simulink model "TST_AirCtl_Gov"  (R2016b)
settings: Solver=FixedStepDiscrete  StartTime=0.0  StopTime=simTime  FixedStep=sampleTime  RelTol=1e-3
values from neighbouring files (symbols this model uses):
  testCase = 1    [initTST_AirCtl_Gov_001.m]
libraries: simulink x6, UnitTest_Lib x4
settings Model: Creator=zhulinfeng  LastModifiedBy=zhulinfeng
settings DebuggingCC: SignalRangeChecking=error

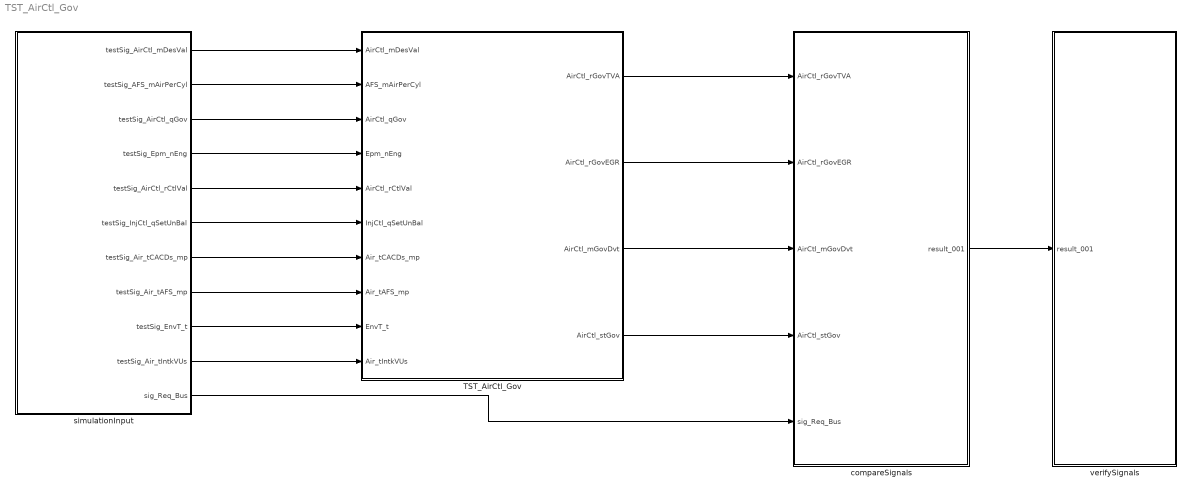
== system TST_AirCtl_Gov ==
  TST_AirCtl_Gov : Subsystem
  compareSignals : Subsystem
  simulationInput : Subsystem
  verifySignals : Subsystem
  wires:
  simulationInput/1(testSig_AirCtl_mDesVal) -> TST_AirCtl_Gov/1(AirCtl_mDesVal)
  simulationInput/2(testSig_AFS_mAirPerCyl) -> TST_AirCtl_Gov/2(AFS_mAirPerCyl)
  simulationInput/3(testSig_AirCtl_qGov) -> TST_AirCtl_Gov/3(AirCtl_qGov)
  simulationInput/4(testSig_Epm_nEng) -> TST_AirCtl_Gov/4(Epm_nEng)
  simulationInput/5(testSig_AirCtl_rCtlVal) -> TST_AirCtl_Gov/5(AirCtl_rCtlVal)
  simulationInput/6(testSig_InjCtl_qSetUnBal) -> TST_AirCtl_Gov/6(InjCtl_qSetUnBal)
  simulationInput/7(testSig_Air_tCACDs_mp) -> TST_AirCtl_Gov/7(Air_tCACDs_mp)
  simulationInput/8(testSig_Air_tAFS_mp) -> TST_AirCtl_Gov/8(Air_tAFS_mp)
  simulationInput/9(testSig_EnvT_t) -> TST_AirCtl_Gov/9(EnvT_t)
  simulationInput/10(testSig_Air_tIntkVUs) -> TST_AirCtl_Gov/10(Air_tIntkVUs)
  TST_AirCtl_Gov/1(AirCtl_rGovTVA) -> compareSignals/1(AirCtl_rGovTVA)
  TST_AirCtl_Gov/2(AirCtl_rGovEGR) -> compareSignals/2(AirCtl_rGovEGR)
  TST_AirCtl_Gov/3(AirCtl_mGovDvt) -> compareSignals/3(AirCtl_mGovDvt)
  TST_AirCtl_Gov/4(AirCtl_stGov) -> compareSignals/4(AirCtl_stGov)
  simulationInput/11(sig_Req_Bus) -> compareSignals/5(sig_Req_Bus)
  compareSignals/1(result_001) -> verifySignals/1(result_001)

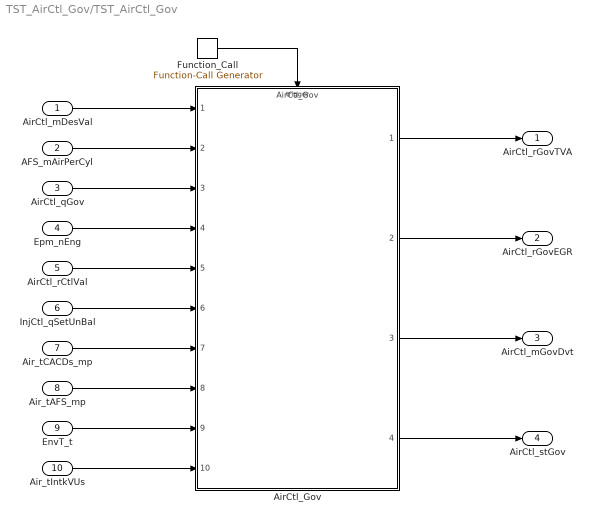
== system TST_AirCtl_Gov/TST_AirCtl_Gov ==
  AirCtl_mDesVal : Inport
  AFS_mAirPerCyl : Inport  Port=2
  AirCtl_qGov : Inport  Port=3
  Epm_nEng : Inport  Port=4
  AirCtl_rCtlVal : Inport  Port=5
  InjCtl_qSetUnBal : Inport  Port=6
  Air_tCACDs_mp : Inport  Port=7
  Air_tAFS_mp : Inport  Port=8
  EnvT_t : Inport  Port=9
  Air_tIntkVUs : Inport  Port=10
  AirCtl_Gov : ModelReference  ModelNameDialog=AirCtl_Gov  SimulationMode=Normal  ModelReferenceVersion=1.96  TriggerPortName=function  TriggerPortTriggerType=function-call  TriggerPortStatesWhenEnabling=held
  Function_Call : simulink/Ports & Subsystems/Function-Call Generator  sample_time=sampleTime  numberOfIterations=1
  AirCtl_rGovTVA : Outport
  AirCtl_rGovEGR : Outport  Port=2
  AirCtl_mGovDvt : Outport  Port=3
  AirCtl_stGov : Outport  Port=4
  wires:
  Function_Call/1 -> AirCtl_Gov/Trigger
  AirCtl_mDesVal/1 -> AirCtl_Gov/1
  AFS_mAirPerCyl/1 -> AirCtl_Gov/2
  AirCtl_qGov/1 -> AirCtl_Gov/3
  Epm_nEng/1 -> AirCtl_Gov/4
  AirCtl_rCtlVal/1 -> AirCtl_Gov/5
  InjCtl_qSetUnBal/1 -> AirCtl_Gov/6
  Air_tCACDs_mp/1 -> AirCtl_Gov/7
  Air_tAFS_mp/1 -> AirCtl_Gov/8
  EnvT_t/1 -> AirCtl_Gov/9
  Air_tIntkVUs/1 -> AirCtl_Gov/10
  AirCtl_Gov/1 -> AirCtl_rGovTVA/1
  AirCtl_Gov/2 -> AirCtl_rGovEGR/1
  AirCtl_Gov/3 -> AirCtl_mGovDvt/1
  AirCtl_Gov/4 -> AirCtl_stGov/1

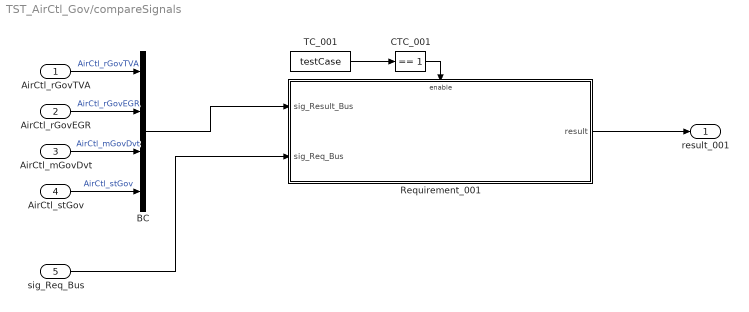
== system TST_AirCtl_Gov/compareSignals ==
  AirCtl_rGovTVA : Inport
  AirCtl_rGovEGR : Inport  Port=2
  AirCtl_mGovDvt : Inport  Port=3
  AirCtl_stGov : Inport  Port=4
  sig_Req_Bus : Inport  Port=5
  BC : BusCreator  Inputs=4
  CTC_001 : simulink/Logic and Bit Operations/Compare To Constant  relop===  const=1  OutDataTypeStr=boolean
  Requirement_001 : Subsystem
  TC_001 : Constant  Value=testCase
  result_001 : Outport
  wires:
  AirCtl_rGovTVA/1 -> BC/1  "AirCtl_rGovTVA"
  AirCtl_rGovEGR/1 -> BC/2  "AirCtl_rGovEGR"
  AirCtl_mGovDvt/1 -> BC/3  "AirCtl_mGovDvt"
  AirCtl_stGov/1 -> BC/4  "AirCtl_stGov"
  TC_001/1 -> CTC_001/1
  CTC_001/1 -> Requirement_001/Enable
  sig_Req_Bus/1 -> Requirement_001/2(sig_Req_Bus)
  BC/1 -> Requirement_001/1(sig_Result_Bus)
  Requirement_001/1(result) -> result_001/1

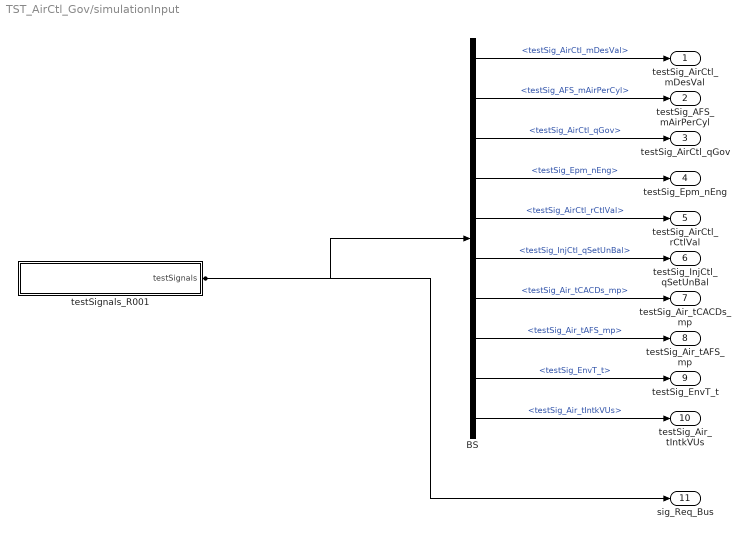
== system TST_AirCtl_Gov/simulationInput ==
  BS : BusSelector  OutputSignals=testSig_AirCtl_mDesVal,testSig_AFS_mAirPerCyl,testSig_AirCtl_qGov,testSig_Epm_nEng,testSig_AirCtl_rCtlVal,testSig_InjCtl_qSetUnBal,testSig_Air_tCACDs_mp,testSig_Air_tAFS_mp,testSig_EnvT_t,testSig_Air_tIntkVUs
  testSignals_R001 : Subsystem
  testSig_AirCtl_mDesVal : Outport
  testSig_AFS_mAirPerCyl : Outport  Port=2
  testSig_AirCtl_qGov : Outport  Port=3
  testSig_Epm_nEng : Outport  Port=4
  testSig_AirCtl_rCtlVal : Outport  Port=5
  testSig_InjCtl_qSetUnBal : Outport  Port=6
  testSig_Air_tCACDs_mp : Outport  Port=7
  testSig_Air_tAFS_mp : Outport  Port=8
  testSig_EnvT_t : Outport  Port=9
  testSig_Air_tIntkVUs : Outport  Port=10
  sig_Req_Bus : Outport  Port=11
  wires:
  BS/1 -> testSig_AirCtl_mDesVal/1  "<testSig_AirCtl_mDesVal>"
  BS/2 -> testSig_AFS_mAirPerCyl/1  "<testSig_AFS_mAirPerCyl>"
  BS/3 -> testSig_AirCtl_qGov/1  "<testSig_AirCtl_qGov>"
  BS/4 -> testSig_Epm_nEng/1  "<testSig_Epm_nEng>"
  BS/5 -> testSig_AirCtl_rCtlVal/1  "<testSig_AirCtl_rCtlVal>"
  BS/6 -> testSig_InjCtl_qSetUnBal/1  "<testSig_InjCtl_qSetUnBal>"
  BS/7 -> testSig_Air_tCACDs_mp/1  "<testSig_Air_tCACDs_mp>"
  BS/8 -> testSig_Air_tAFS_mp/1  "<testSig_Air_tAFS_mp>"
  BS/9 -> testSig_EnvT_t/1  "<testSig_EnvT_t>"
  BS/10 -> testSig_Air_tIntkVUs/1  "<testSig_Air_tIntkVUs>"
  testSignals_R001/1(testSignals) -> BS/1, sig_Req_Bus/1

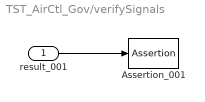
== system TST_AirCtl_Gov/verifySignals ==
  result_001 : Inport
  Assertion_001 : Assertion  Enabled=off
  wires:
  result_001/1 -> Assertion_001/1

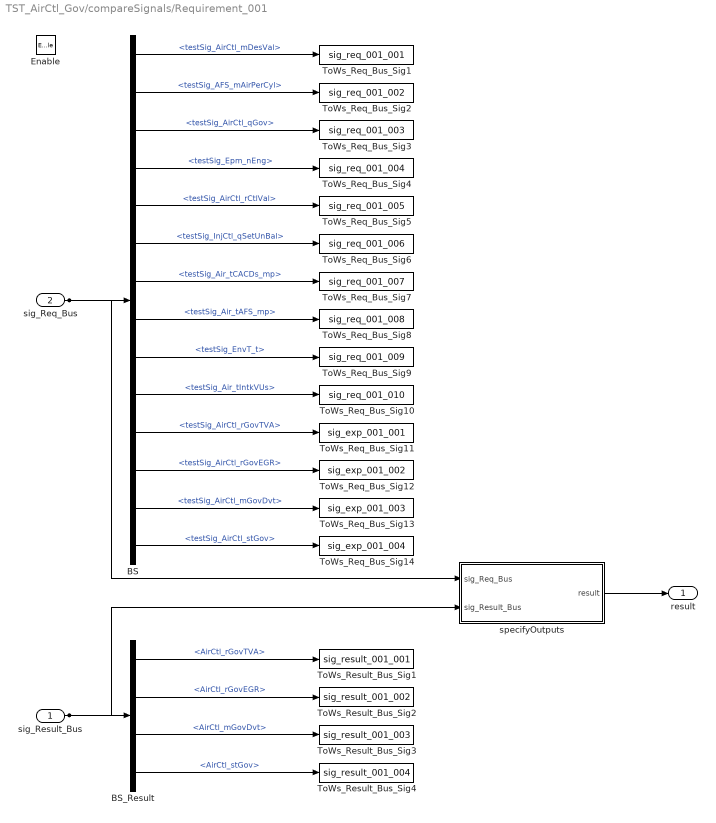
== system TST_AirCtl_Gov/compareSignals/Requirement_001 ==
  sig_Result_Bus : Inport
  sig_Req_Bus : Inport  Port=2
  Enable : EnablePort
  BS : BusSelector  OutputSignals=testSig_AirCtl_mDesVal,testSig_AFS_mAirPerCyl,testSig_AirCtl_qGov,testSig_Epm_nEng,testSig_AirCtl_rCtlVal,testSig_InjCtl_qSetUnBal,testSig_Air_tCACDs_mp,testSig_Air_tAFS_mp,testSig_EnvT_t,testSig_Air_tIntkVUs,testSig_AirCtl_rGovTVA,testSig_AirCtl_rGovEGR,testSig_AirCtl_mGovDvt,testSig_AirCtl_stGov
  BS_Result : BusSelector  OutputSignals=AirCtl_rGovTVA,AirCtl_rGovEGR,AirCtl_mGovDvt,AirCtl_stGov
  ToWs_Req_Bus_Sig1 : ToWorkspace  VariableName=sig_req_001_001  SaveFormat=Structure With Time
  ToWs_Req_Bus_Sig10 : ToWorkspace  VariableName=sig_req_001_010  SaveFormat=Structure With Time
  ToWs_Req_Bus_Sig11 : ToWorkspace  VariableName=sig_exp_001_001  SaveFormat=Structure With Time
  ToWs_Req_Bus_Sig12 : ToWorkspace  VariableName=sig_exp_001_002  SaveFormat=Structure With Time
  ToWs_Req_Bus_Sig13 : ToWorkspace  VariableName=sig_exp_001_003  SaveFormat=Structure With Time
  ToWs_Req_Bus_Sig14 : ToWorkspace  VariableName=sig_exp_001_004  SaveFormat=Structure With Time
  ToWs_Req_Bus_Sig2 : ToWorkspace  VariableName=sig_req_001_002  SaveFormat=Structure With Time
  ToWs_Req_Bus_Sig3 : ToWorkspace  VariableName=sig_req_001_003  SaveFormat=Structure With Time
  ToWs_Req_Bus_Sig4 : ToWorkspace  VariableName=sig_req_001_004  SaveFormat=Structure With Time
  ToWs_Req_Bus_Sig5 : ToWorkspace  VariableName=sig_req_001_005  SaveFormat=Structure With Time
  ToWs_Req_Bus_Sig6 : ToWorkspace  VariableName=sig_req_001_006  SaveFormat=Structure With Time
  ToWs_Req_Bus_Sig7 : ToWorkspace  VariableName=sig_req_001_007  SaveFormat=Structure With Time
  ToWs_Req_Bus_Sig8 : ToWorkspace  VariableName=sig_req_001_008  SaveFormat=Structure With Time
  ToWs_Req_Bus_Sig9 : ToWorkspace  VariableName=sig_req_001_009  SaveFormat=Structure With Time
  ToWs_Result_Bus_Sig1 : ToWorkspace  VariableName=sig_result_001_001  SaveFormat=Structure With Time
  ToWs_Result_Bus_Sig2 : ToWorkspace  VariableName=sig_result_001_002  SaveFormat=Structure With Time
  ToWs_Result_Bus_Sig3 : ToWorkspace  VariableName=sig_result_001_003  SaveFormat=Structure With Time
  ToWs_Result_Bus_Sig4 : ToWorkspace  VariableName=sig_result_001_004  SaveFormat=Structure With Time
  specifyOutputs : Subsystem
  result : Outport
  wires:
  sig_Req_Bus/1 -> BS/1, specifyOutputs/1(sig_Req_Bus)
  BS/1 -> ToWs_Req_Bus_Sig1/1  "<testSig_AirCtl_mDesVal>"
  BS/2 -> ToWs_Req_Bus_Sig2/1  "<testSig_AFS_mAirPerCyl>"
  BS/3 -> ToWs_Req_Bus_Sig3/1  "<testSig_AirCtl_qGov>"
  BS/4 -> ToWs_Req_Bus_Sig4/1  "<testSig_Epm_nEng>"
  BS/5 -> ToWs_Req_Bus_Sig5/1  "<testSig_AirCtl_rCtlVal>"
  BS/6 -> ToWs_Req_Bus_Sig6/1  "<testSig_InjCtl_qSetUnBal>"
  BS/7 -> ToWs_Req_Bus_Sig7/1  "<testSig_Air_tCACDs_mp>"
  BS/8 -> ToWs_Req_Bus_Sig8/1  "<testSig_Air_tAFS_mp>"
  BS/9 -> ToWs_Req_Bus_Sig9/1  "<testSig_EnvT_t>"
  BS/10 -> ToWs_Req_Bus_Sig10/1  "<testSig_Air_tIntkVUs>"
  BS/11 -> ToWs_Req_Bus_Sig11/1  "<testSig_AirCtl_rGovTVA>"
  BS/12 -> ToWs_Req_Bus_Sig12/1  "<testSig_AirCtl_rGovEGR>"
  BS/13 -> ToWs_Req_Bus_Sig13/1  "<testSig_AirCtl_mGovDvt>"
  BS/14 -> ToWs_Req_Bus_Sig14/1  "<testSig_AirCtl_stGov>"
  sig_Result_Bus/1 -> BS_Result/1, specifyOutputs/2(sig_Result_Bus)
  BS_Result/1 -> ToWs_Result_Bus_Sig1/1  "<AirCtl_rGovTVA>"
  BS_Result/2 -> ToWs_Result_Bus_Sig2/1  "<AirCtl_rGovEGR>"
  BS_Result/3 -> ToWs_Result_Bus_Sig3/1  "<AirCtl_mGovDvt>"
  BS_Result/4 -> ToWs_Result_Bus_Sig4/1  "<AirCtl_stGov>"
  specifyOutputs/1(result) -> result/1

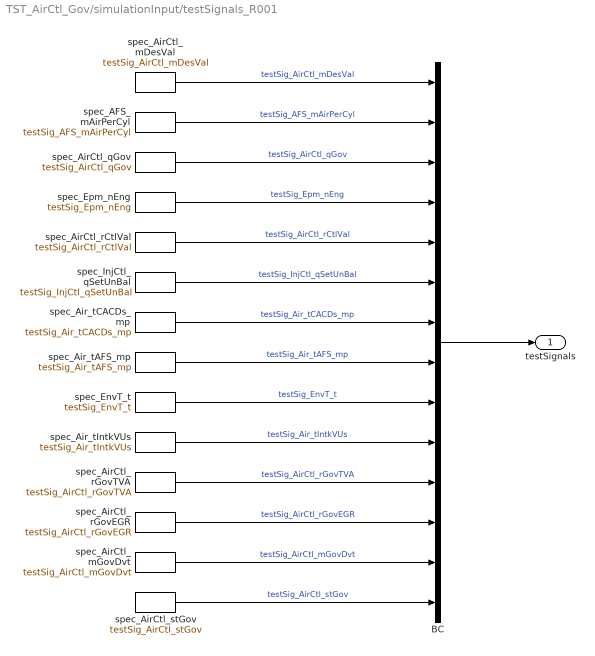
== system TST_AirCtl_Gov/simulationInput/testSignals_R001 ==
  BC : BusCreator  Inputs=14
  spec_AFS_mAirPerCyl : FromWorkspace  VariableName=testSig_AFS_mAirPerCyl  Interpolate=off  OutputAfterFinalValue=Holding final value
  spec_AirCtl_mDesVal : FromWorkspace  VariableName=testSig_AirCtl_mDesVal  Interpolate=off  OutputAfterFinalValue=Holding final value
  spec_AirCtl_mGovDvt : FromWorkspace  VariableName=testSig_AirCtl_mGovDvt  Interpolate=off  OutputAfterFinalValue=Holding final value
  spec_AirCtl_qGov : FromWorkspace  VariableName=testSig_AirCtl_qGov  Interpolate=off  OutputAfterFinalValue=Holding final value
  spec_AirCtl_rCtlVal : FromWorkspace  VariableName=testSig_AirCtl_rCtlVal  Interpolate=off  OutputAfterFinalValue=Holding final value
  spec_AirCtl_rGovEGR : FromWorkspace  VariableName=testSig_AirCtl_rGovEGR  Interpolate=off  OutputAfterFinalValue=Holding final value
  spec_AirCtl_rGovTVA : FromWorkspace  VariableName=testSig_AirCtl_rGovTVA  Interpolate=off  OutputAfterFinalValue=Holding final value
  spec_AirCtl_stGov : FromWorkspace  VariableName=testSig_AirCtl_stGov  Interpolate=off  OutputAfterFinalValue=Holding final value
  spec_Air_tAFS_mp : FromWorkspace  VariableName=testSig_Air_tAFS_mp  Interpolate=off  OutputAfterFinalValue=Holding final value
  spec_Air_tCACDs_mp : FromWorkspace  VariableName=testSig_Air_tCACDs_mp  Interpolate=off  OutputAfterFinalValue=Holding final value
  spec_Air_tIntkVUs : FromWorkspace  VariableName=testSig_Air_tIntkVUs  Interpolate=off  OutputAfterFinalValue=Holding final value
  spec_EnvT_t : FromWorkspace  VariableName=testSig_EnvT_t  Interpolate=off  OutputAfterFinalValue=Holding final value
  spec_Epm_nEng : FromWorkspace  VariableName=testSig_Epm_nEng  Interpolate=off  OutputAfterFinalValue=Holding final value
  spec_InjCtl_qSetUnBal : FromWorkspace  VariableName=testSig_InjCtl_qSetUnBal  Interpolate=off  OutputAfterFinalValue=Holding final value
  testSignals : Outport
  wires:
  BC/1 -> testSignals/1
  spec_AirCtl_mDesVal/1 -> BC/1  "testSig_AirCtl_mDesVal"
  spec_AFS_mAirPerCyl/1 -> BC/2  "testSig_AFS_mAirPerCyl"
  spec_AirCtl_qGov/1 -> BC/3  "testSig_AirCtl_qGov"
  spec_Epm_nEng/1 -> BC/4  "testSig_Epm_nEng"
  spec_AirCtl_rCtlVal/1 -> BC/5  "testSig_AirCtl_rCtlVal"
  spec_InjCtl_qSetUnBal/1 -> BC/6  "testSig_InjCtl_qSetUnBal"
  spec_Air_tCACDs_mp/1 -> BC/7  "testSig_Air_tCACDs_mp"
  spec_Air_tAFS_mp/1 -> BC/8  "testSig_Air_tAFS_mp"
  spec_EnvT_t/1 -> BC/9  "testSig_EnvT_t"
  spec_Air_tIntkVUs/1 -> BC/10  "testSig_Air_tIntkVUs"
  spec_AirCtl_rGovTVA/1 -> BC/11  "testSig_AirCtl_rGovTVA"
  spec_AirCtl_rGovEGR/1 -> BC/12  "testSig_AirCtl_rGovEGR"
  spec_AirCtl_mGovDvt/1 -> BC/13  "testSig_AirCtl_mGovDvt"
  spec_AirCtl_stGov/1 -> BC/14  "testSig_AirCtl_stGov"

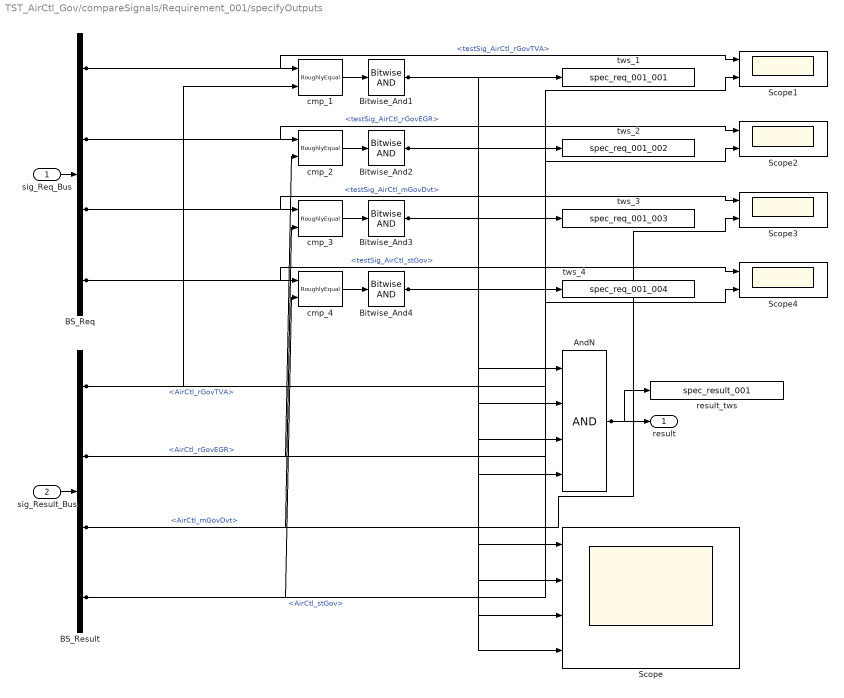
== system TST_AirCtl_Gov/compareSignals/Requirement_001/specifyOutputs ==
  sig_Req_Bus : Inport
  sig_Result_Bus : Inport  Port=2
  AndN : Logic  Inputs=4
  BS_Req : BusSelector  OutputSignals=testSig_AirCtl_rGovTVA,testSig_AirCtl_rGovEGR,testSig_AirCtl_mGovDvt,testSig_AirCtl_stGov
  BS_Result : BusSelector  OutputSignals=AirCtl_rGovTVA,AirCtl_rGovEGR,AirCtl_mGovDvt,AirCtl_stGov
  Bitwise_And{1..4} (4 alike) : simulink/Logic and Bit Operations/Bitwise Operator  logicop=AND  UseBitMask=off  BitMask=bin2dec('11011001')  BitMaskRealWorld=Stored Integer
  Scope : Scope  NumInputPorts=4
  Scope{1..4} (4 alike) : Scope  NumInputPorts=2
  cmp_{1..4} (4 alike) : UnitTest_Lib/RoughlyEqual  slope=0.1
  result_tws : ToWorkspace  VariableName=spec_result_001
  tws_1 : ToWorkspace  VariableName=spec_req_001_001
  tws_2 : ToWorkspace  VariableName=spec_req_001_002
  tws_3 : ToWorkspace  VariableName=spec_req_001_003
  tws_4 : ToWorkspace  VariableName=spec_req_001_004
  result : Outport
  wires:
  sig_Req_Bus/1 -> BS_Req/1
  sig_Result_Bus/1 -> BS_Result/1
  AndN/1 -> result/1, result_tws/1
  BS_Req/1 -> cmp_1/1, Scope1/1  "<testSig_AirCtl_rGovTVA>"
  BS_Result/1 -> cmp_1/2, Scope1/2  "<AirCtl_rGovTVA>"
  cmp_1/1 -> Bitwise_And1/1
  Bitwise_And1/1 -> tws_1/1, AndN/1, Scope/1
  BS_Req/2 -> cmp_2/1, Scope2/1  "<testSig_AirCtl_rGovEGR>"
  BS_Result/2 -> cmp_2/2, Scope2/2  "<AirCtl_rGovEGR>"
  cmp_2/1 -> Bitwise_And2/1
  Bitwise_And2/1 -> tws_2/1, AndN/2, Scope/2
  BS_Req/3 -> cmp_3/1, Scope3/1  "<testSig_AirCtl_mGovDvt>"
  BS_Result/3 -> cmp_3/2, Scope3/2  "<AirCtl_mGovDvt>"
  cmp_3/1 -> Bitwise_And3/1
  Bitwise_And3/1 -> tws_3/1, AndN/3, Scope/3
  BS_Req/4 -> cmp_4/1, Scope4/1  "<testSig_AirCtl_stGov>"
  BS_Result/4 -> cmp_4/2, Scope4/2  "<AirCtl_stGov>"
  cmp_4/1 -> Bitwise_And4/1
  Bitwise_And4/1 -> tws_4/1, AndN/4, Scope/4
